simulink model "robotSafeTrajectoryTracking"  (R2024a)
settings: Solver=FixedStepAuto  StartTime=0.0  StopTime=20  FixedStep=0.005  RelTol=1e-3
PostLoadFcn:
  | % load sawyer robot mesh for visualization
  | exampleHelperLoadSawyerMesh()
InitFcn:
  | objectPos = 0.6;
  | refPos = 0.185;
StartFcn:
  | objectPos = 0.6;
model workspace (MAT data in the model file):
  p = [0 0 0 0 0 0 0.0291358024691 -0.218518518519 0.437037037037 0 0 -1.18 ... (42 elements, 6x7)]
  q0 = [0; -1.18; 0; 2.18; 0; -1.0008; 3.3161]
  q1 = [0; 0; 0; 0; 0; 0; 0]
  sawyer : robotics.RigidBodyTree (value not decoded)
  tDuration = 3
  tStart = 0.5
undefined symbols (not defined in the file or in its folder): endeffectorPos_sm, endeffectorVel_sm, objectPos_sm, reactionForce_sm, torque_input1_sm, torque_input2_sm, torque_input3_sm, torque_input4_sm, torque_input5_sm, torque_input6_sm, torque_input7_sm, X, Y, Z
libraries: sm_lib x153, nesl_utility x33, robotmaniplib x5, robotcorelib x2
(part 4 of 4)

== matlab function robotSafeTrajectoryTracking/Simscape Model with Simple Contact Mechanics/MATLAB Function5 ==
  data: singleValue input
function writeToWorkspace(singleValue)
    % Write the input value to a workspace variable
    assignin('base', 'torque_input6_sm', singleValue);
end

== matlab function robotSafeTrajectoryTracking/Simscape Model with Simple Contact Mechanics/MATLAB Function6 ==
  data: singleValue input
function writeToWorkspace(singleValue)
    % Write the input value to a workspace variable
    assignin('base', 'torque_input7_sm', singleValue);
end

== matlab function robotSafeTrajectoryTracking/Simscape Model with Simple Contact Mechanics/MATLAB Function7 ==
  data: singleValue input
function writeToWorkspace(singleValue)
    % Write the input value to a workspace variable
    assignin('base', 'endeffectorPos_sm', singleValue);
end

== matlab function robotSafeTrajectoryTracking/Simscape Model with Simple Contact Mechanics/MATLAB Function8 ==
  data: singleValue input
function writeToWorkspace(singleValue)
    % Write the input value to a workspace variable
    assignin('base', 'endeffectorVel_sm', singleValue);
end

== matlab function robotSafeTrajectoryTracking/Simscape Model with Simple Contact Mechanics/MATLAB Function9 ==
  data: singleValue input
function writeToWorkspace(singleValue)
    % Write the input value to a workspace variable
    assignin('base', 'objectPos_sm', singleValue);
end

== matlab function robotSafeTrajectoryTracking/Simscape Model with Simple Contact Mechanics/MATLAB Function10 ==
  data: singleValue input
function writeToWorkspace(singleValue)
    % Write the input value to a workspace variable
    assignin('base', 'reactionForce_sm', singleValue);
end
